simulink model "controlGPI_pos_2dof_sinMI"  (R2023b)
settings: Solver=ode45  StartTime=0.0  StopTime=tsim  FixedStep=5e-4  MaxStep=tstep
undefined symbols (not defined in the file): contr_robot_params, ddq, dq, ndof, NN_Bspline_params, NN_RBF_params, nn_select, Pc, q, q0, q_cero, q_eq, robot_params, t_qeq_init, t_tr_init, t_trtr, tau_L, tau_L_mags, tr_muestra, Wc, Zc
libraries: simulink x2
(part 2 of 2)

== matlab function controlGPI_pos_2dof_sinMI/ControladorGPI + NN/Ley de control ==
  data: robot_din input; v output size=[2,1]; eqB5 input size=[2,1]; eqB4 input size=[2,1]; eqB3 input size=[2,1]; eqB2 input size=[2,1]; eqB1 input size=[2,1]; tau_R output size=[2,1]
function [v,tau_R] = fcn(robot_din,eqB5,eqB4,eqB3,eqB2,eqB1)

D = robot_din.D;

v = - eqB5 - eqB4 - eqB3 - eqB2 - eqB1;

tau_R = D*v;

== matlab function controlGPI_pos_2dof_sinMI/ControladorGPI + NN/Red neuronal/B-Spline NNs/Red Neuronal B-spline ==
  data: NN_Bspline_params input; e_q input size=[2,1]; Wc output size=[2,1]; Zc output size=[2,1]; Pc output size=[2,1]; e_px input size=[2,1]; e_py input size=[2,1]; newweightsWc output; newweightsZc output; newweightsPc output; weightsWc input; weightsZc input; weightsPc input
function [Wc, Zc, Pc, newweightsWc, newweightsZc, newweightsPc]   = BSpline_NN(NN_Bspline_params,e_q,e_px,e_py,weightsWc,weightsZc,weightsPc)

deltaWc = NN_Bspline_params.delta.deltaWc;
deltaZc = NN_Bspline_params.delta.deltaZc;
deltaPc = NN_Bspline_params.delta.deltaPc;

lambdaWc = NN_Bspline_params.lambda.lambdaWc;
lambdaZc = NN_Bspline_params.lambda.lambdaZc;
lambdaPc = NN_Bspline_params.lambda.lambdaPc;

if NN_Bspline_params.num_inputs == 1
    nn_inputs = e_q;
elseif NN_Bspline_params.num_inputs == 3
    nn_inputs = [e_q,e_px,e_py];
else
    nn_inputs = e_q;
end

delta = [deltaWc;
         deltaZc;
         deltaPc];

lambda = cat(1,lambdaWc,lambdaZc,lambdaPc);
weights = cat(1,weightsWc,weightsZc,weightsPc);

[newparams,newweights] = NN_Bspline.Gradient_Descent(delta,weights,lambda,nn_inputs);

Wc = newparams(1,:)';
Zc = newparams(2,:)';
Pc = newparams(3,:)';

newweightsWc = newweights(1,:,:);
newweightsZc = newweights(2,:,:);
newweightsPc = newweights(3,:,:);

end

== matlab function controlGPI_pos_2dof_sinMI/ControladorGPI + NN/Red neuronal/RBF NNs/Red Neuronal RBF ==
  data: NN_RBF_params input; e_q input size=[2,1]; Wc output size=[2,1]; Zc output size=[2,1]; Pc output size=[2,1]; e_px input size=[2,1]; e_py input size=[2,1]; weightsWc output; weightsZc output; weightsPc output; weightsWc input; weightsZc input; weightsPc input
function [Wc, Zc, Pc, weightsWc, weightsZc, weightsPc] = RBF_NN(NN_RBF_params,e_q,e_px,e_py, weightsWc, weightsZc, weightsPc)

%k = NN_RBF_params.rbf_params.k;
centers = NN_RBF_params.rbf_params.C';
radius = NN_RBF_params.rbf_params.sigma;

deltaWc = NN_RBF_params.delta.deltaWc;
deltaZc = NN_RBF_params.delta.deltaZc;
deltaPc = NN_RBF_params.delta.deltaPc;

if NN_RBF_params.num_inputs == 1
    NNRBF_inputs = e_q;
elseif NN_RBF_params.num_inputs == 3
    NNRBF_inputs = [e_q,e_px,e_py];
else
    NNRBF_inputs = e_q;
end

delta = [deltaWc;
         deltaZc;
         deltaPc];

weights = cat(1,weightsWc,weightsZc,weightsPc);

[newparams,newweights] = NN_RBF.Gradient_Descent(delta,weights,centers,radius,NNRBF_inputs);

Wc = newparams(1,:)';
Zc = newparams(2,:)';
Pc = newparams(3,:)';

weightsWc = newweights(1,:,:);
weightsZc = newweights(2,:,:);
weightsPc = newweights(3,:,:);

end

== matlab function controlGPI_pos_2dof_sinMI/ControladorGPI + NN/Matriz de parámetros B ==
  data: B5 output size=[2,1]; B4 output size=[2,1]; B3 output size=[2,1]; B2 output size=[2,1]; Zc input size=[2,1]; B1 output size=[2,1]; Wc input size=[2,1]; Pc input size=[2,1]
function [B5,B4,B3,B2,B1] = fcn(Zc,Wc,Pc)

B = zeros(2,6);

B(:,1) = Wc.^4.*Pc;
B(:,2) = 4*Wc.^3.*Zc.*Pc + Wc.^4;
B(:,3) = 4*Wc.^3.*Zc + 4*Wc.^2.*Zc.^2.*Pc + 2.*Wc.^2.*Pc;
B(:,4) = 2*Wc.^2 + 4*Wc.^2.*Zc.^2 + 4*Wc.*Zc.*Pc;
B(:,5) = 4*Wc.*Zc + Pc;
% B(:,6) = ones(3,6);

B1 = B(:,1);
B2 = B(:,2);
B3 = B(:,3);
B4 = B(:,4);
B5 = B(:,5);
% B6 = B(:,6);

== matlab function controlGPI_pos_2dof_sinMI/q to xyz (robot)/q to xyz (referencia) ==
  data: p output size=[2,2]; robot_params input; q input size=[2,1]; dq input size=[2,1]; ddq input size=[2,1]; dp output size=[2,1]; ddp output size=[2,1]
function [p,dp,ddp] = fcn(robot_params,q,dq,ddq)

[p,dp,ddp] = robot_cin.cin_dir_2dof(robot_params,q,dq,ddq);

== matlab function controlGPI_pos_2dof_sinMI/Trayectoria de referencia/Dinamica inversa (referencia) ==
  data: robot_params input; tau_s output size=[2,1]; q input size=[2,1]; dq input size=[2,1]; ddq input size=[2,1]
function tau_s = fcn(robot_params,q,dq,ddq)

robot_din = robot_dinm.din_2dof(robot_params,q,dq);

D = robot_din.D;
C = robot_din.C;
G = robot_din.G;
g = robot_din.g;

tau_s = D*ddq + C*dq + G*g;

== matlab function controlGPI_pos_2dof_sinMI/Trayectoria de referencia/Inicializar posición de robot manipulador/interp_pol7_q_r ==
  data: t input; q_eq input; interp_qpos output; q_cero input; q_tr_init input; t0 input; t1 input; t_trtr input; tr_muestra input; ndof input
function interp_qpos = fcn(t,q_eq,q_cero,q_tr_init,t0,t1,t_trtr,tr_muestra,ndof)

tcero = t0/2 + t1/2;

if t < tcero
    dist1 = norm(zeros(size(q_eq)) - q_eq);
    
    if dist1 > 0
        qpol1 = pol7(t,0,dist1,t0,tcero);
        dire1 = (zeros(size(q_eq)) - q_eq)/dist1;
        
        interp_qpos = q_eq + dire1*qpol1;
    else
        interp_qpos = q_eq;
    end
elseif t >= tcero && t < t1
    dist2 = norm(q_cero - zeros(size(q_eq)));
    if dist2 > 0
        qpol2 = pol7(t,0,dist2,tcero,t1);
        dire2 = (q_cero - zeros(size(q_eq)))/dist2;
    
        interp_qpos =  zeros(size(q_eq)) + dire2*qpol2;
    else
        interp_qpos = zeros(size(q_eq));
    end
elseif t >= t1 && t < t1 + t_trtr
    if (tr_muestra == 1 || ndof ~= 6) && ndof ~= 2
        dist3 = norm(q_tr_init - q_cero);
        if dist3 > 0
            qpol3 = pol7(t,0,dist3,t1,t1 + t_trtr);
            dire3 = (q_tr_init - q_cero)/dist3;
            
            interp_qpos =  q_cero + dire3*qpol3;
        else
            interp_qpos = q_cero;
        end
    else
        interp_qpos = q_tr_init;
    end
elseif t >= t1 + t_trtr
    interp_qpos = q_tr_init;
else
    interp_qpos = q_eq;
end

== matlab function controlGPI_pos_2dof_sinMI/Norm e_q ==
  data: u input; y output
function y = norm(u)

y = norm(u,2);

== matlab function controlGPI_pos_2dof_sinMI/Trayectoria de referencia/q to xyz (referencia) ==
  data: p output size=[2,2]; robot_params input; q input size=[2,1]; dq input; ddq input; dp output; ddp output
function [p,dp,ddp] = fcn(robot_params,q,dq,ddq)

[p,dp,ddp] = robot_cin.cin_dir_2dof(robot_params,q,dq,ddq);
